simulink model "trajectory_sim"  (R2021b)
settings: Solver=ode4  StartTime=TIME.Start  StopTime=TIME.Final  FixedStep=TIME.Ts  RelTol=1e-3
values from neighbouring files (symbols this model uses):
  Ax = 0.0    (= 0)    [Vehicle_exmaple.m]    (also in main_trajectory.m)
  Ay = -9.81    [Vehicle_exmaple.m]    (also in main_trajectory.m)
  POS0 = [0, 0]    [main_trajectory.m]
  TIME = struct('Ts'   , 1e-3,                'Start', 0.0 ,                'Final', 0.0 ,                'idx'   ,1   )    [trajectory_simulation.m]
  Vx0 = V*cos(angle)    [main_trajectory.m]
  Vy0 = V*sin(angle)    [main_trajectory.m]
settings Model: Creator=jinkwak  LastModifiedBy=jinkwak

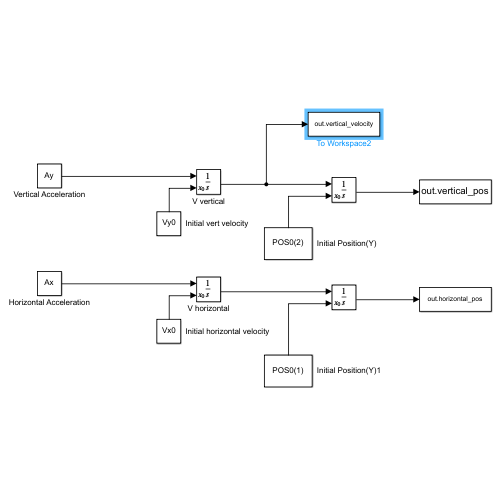
[thumbnail: Simulink's stored preview of the top-level diagram]
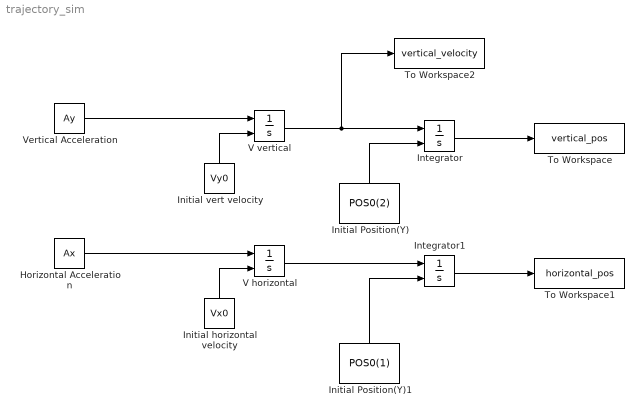
== system trajectory_sim ==
  Horizontal Acceleration : Constant  Value=Ax  SampleTime=TIME.Ts
  Initial Position(Y) : Constant  Value=POS0(2)  SampleTime=TIME.Ts
  Initial Position(Y)1 : Constant  Value=POS0(1)  SampleTime=TIME.Ts
  Initial horizontal velocity : Constant  Value=Vx0  SampleTime=TIME.Ts
  Initial vert velocity : Constant  Value=Vy0  SampleTime=TIME.Ts
  Integrator : Integrator  InitialConditionSource=external
  Integrator1 : Integrator  InitialConditionSource=external
  To Workspace : ToWorkspace  VariableName=vertical_pos  SampleTime=TIME.Ts
      settings: Save2DSignal=2-D array (concatenate along first dimension)
  To Workspace1 : ToWorkspace  VariableName=horizontal_pos  SampleTime=TIME.Ts
      settings: Save2DSignal=2-D array (concatenate along first dimension)
  To Workspace2 : ToWorkspace  VariableName=vertical_velocity  SampleTime=TIME.Ts
      settings: Save2DSignal=2-D array (concatenate along first dimension)
  V horizontal : Integrator  InitialConditionSource=external
  V vertical : Integrator  InitialConditionSource=external
  Vertical Acceleration : Constant  Value=Ay  SampleTime=TIME.Ts
  wires:
  Initial vert velocity/1 -> V vertical/2
  Initial horizontal velocity/1 -> V horizontal/2
  Vertical Acceleration/1 -> V vertical/1
  Horizontal Acceleration/1 -> V horizontal/1
  V vertical/1 -> To Workspace2/1, Integrator/1
  V horizontal/1 -> Integrator1/1
  Initial Position(Y)/1 -> Integrator/2
  Initial Position(Y)1/1 -> Integrator1/2
  Integrator/1 -> To Workspace/1
  Integrator1/1 -> To Workspace1/1
